simulink subsystem "CircuitBreaker"  (R2023b)
settings: Solver=VariableStepAuto  StartTime=0.0  StopTime=10.0  RelTol=1e-3
libraries: spsThreePhaseBreakerLib x1, dspnetwork x1
settings Model: Creator=javiersanderios  LastModifiedBy=javiersanderios

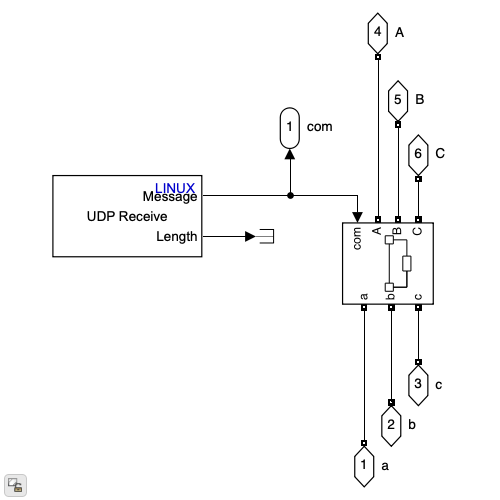
[thumbnail: Simulink's stored preview of the top-level diagram]
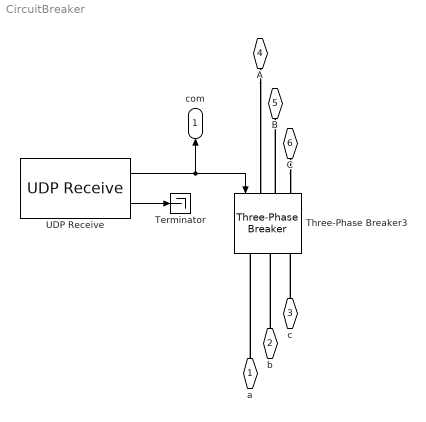
== system CircuitBreaker ==
  Terminator : Terminator
  Three-Phase Breaker3 : spsThreePhaseBreakerLib/Three-Phase Breaker  InitialState=closed  SwitchA=on  SwitchB=on  SwitchC=on  SwitchTimes=[0.2]  External=on  BreakerResistance=0.01  SnubberResistance=1e6  SnubberCapacitance=inf  Measurements=Breaker voltages and currents
  UDP Receive : dspnetwork/UDP Receive  localURL='0.0.0.0'  localPort=30000  remoteURL='0.0.0.0'  remotePort=-1  recvBufferSize=2  dims=1  signalDatatype=uint16  isComplex=off  isVarSize=off  showBlockingTime=on  blockingTime=0  sampletime=0.1  blockPlatform=LINUX
  a : PMIOPort  Side=Left
  b : PMIOPort  Port=2  Side=Left
  c : PMIOPort  Port=3  Side=Left
  A : PMIOPort  Port=4  Side=Right
  B : PMIOPort  Port=5  Side=Right
  C : PMIOPort  Port=6  Side=Right
  com : Outport
  wires:
  UDP Receive/1 -> com/1, Three-Phase Breaker3/1
  UDP Receive/2 -> Terminator/1
  connections:
  b/RConn1 -- Three-Phase Breaker3/RConn2
  c/RConn1 -- Three-Phase Breaker3/RConn3
  A/RConn1 -- Three-Phase Breaker3/LConn1
  Three-Phase Breaker3/LConn2 -- B/RConn1
  C/RConn1 -- Three-Phase Breaker3/LConn3
  a/RConn1 -- Three-Phase Breaker3/RConn1
